simulink model "drivePMSM"  (R2024b)
settings: Solver=VariableStepAuto  StartTime=0.0  StopTime=0.5  MaxStep=1e-3  RelTol=1e-3
undefined symbols (not defined in the file or in its folder): contr_D, contr_Q, contr_Speed, inverter, mot
libraries: simulink x13
settings Model: Creator=giulio  LastModifiedBy=giulio

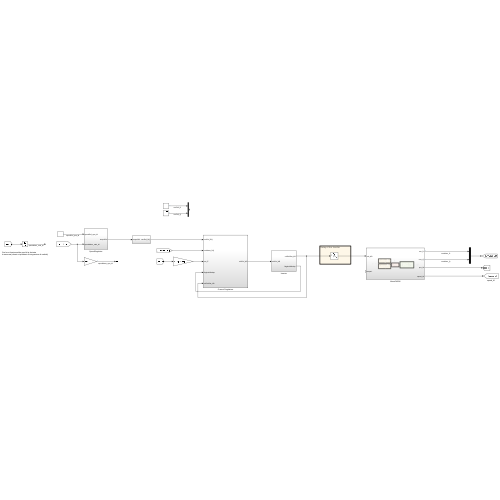
[thumbnail: Simulink's stored preview of the top-level diagram]
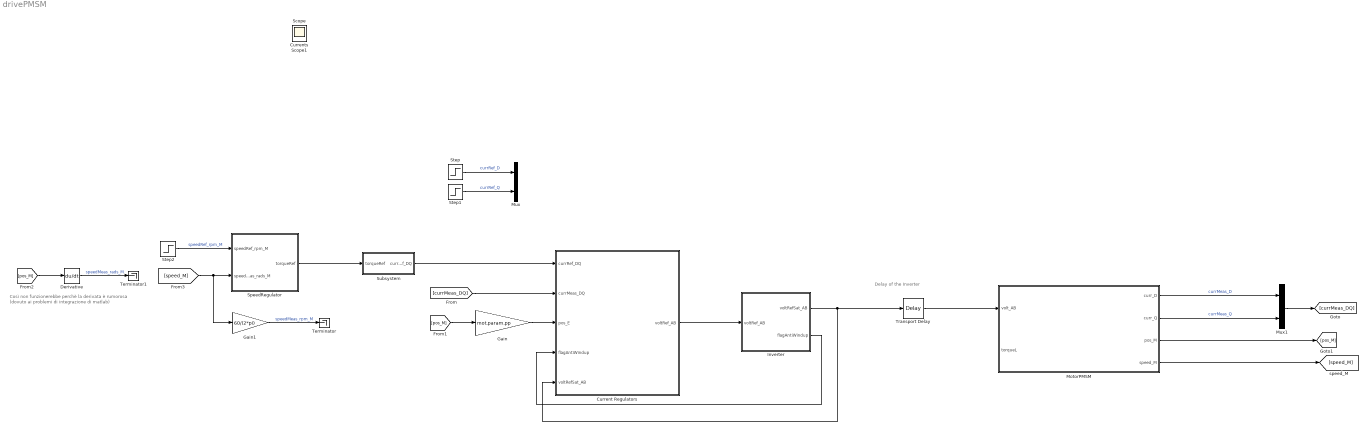
== system drivePMSM ==
  note: Così non funzionerebbe perchè la derivata
      | è rumorosa (dovuto ai problemi di integrazione di matlab)
  note: Delay of the Inverter
  Current Regulators : Subsystem
  Derivative : Derivative
  Gain : Gain  Gain=mot.param.pp
  Gain1 : Gain  Gain=60/(2*pi)
  Inverter : Subsystem
  MotorPMSM : Subsystem
  Mux : Mux  Inputs=2
  Mux1 : Mux  Inputs=2
  SpeedRegulator : Subsystem
  Step : Step  Time=1e-3  SampleTime=0
  Step1 : Step  Time=5e-3  SampleTime=0
  Step2 : Step  Time=0.01  After=0.25*mot.rated.speed_rpm  SampleTime=0
  Subsystem : Subsystem
  Terminator : Terminator
  Terminator1 : Terminator
  Transport Delay : TransportDelay  DelayTime=1.5*inverter.param.timePWM
  Currents : Scope
  Scope : Scope
  Scope1 : Scope
  wires:
  Transport Delay/1 -> MotorPMSM/1(volt_AB)
  Current Regulators/1(voltRef_AB) -> Inverter/1(voltRef_AB)
  Step/1 -> Mux/1  "currRef_D"
  Step1/1 -> Mux/2  "currRef_Q"
  Mux1/1 -> [currMeas_DQ]
  MotorPMSM/1(curr_D) -> Mux1/1  "currMeas_D"
  MotorPMSM/2(curr_Q) -> Mux1/2  "currMeas_Q"
  MotorPMSM/3(pos_M) -> [pos_M]
  [pos_M] -> Gain/1
  Gain/1 -> Current Regulators/3(pos_E)
  Inverter/2(flagAntiWindup) -> Current Regulators/4(flagAntiWindup)
  [currMeas_DQ] -> Current Regulators/2(currMeas_DQ)
  Inverter/1(voltRefSat_AB) -> Current Regulators/5(voltRefSat_AB), Transport Delay/1
  SpeedRegulator/1(torqueRef) -> Subsystem/1(torqueRef)
  Subsystem/1(currRef_DQ) -> Current Regulators/1(currRef_DQ)
  [pos_M] -> Derivative/1
  Step2/1 -> SpeedRegulator/1(speedRef_rpm_M)  "speedRef_rpm_M"
  Gain1/1 -> Terminator/1  "speedMeas_rpm_M"
  MotorPMSM/4(speed_M) -> [speed_M]
  [speed_M] -> Gain1/1, SpeedRegulator/2(speedMeas_rads_M)
  Derivative/1 -> Terminator1/1  "speedMeas_rads_M"

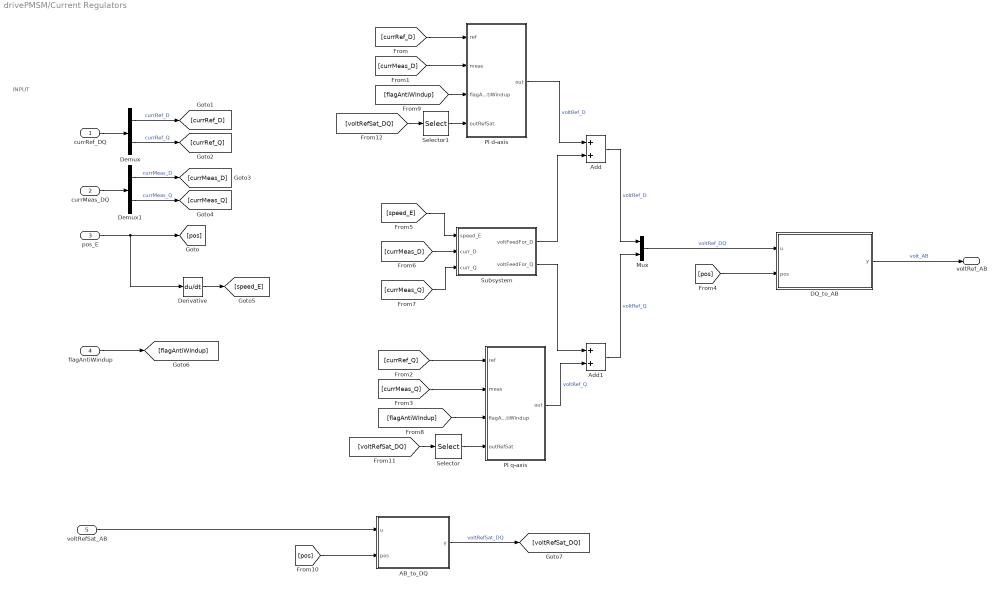
== system drivePMSM/Current Regulators ==
  note: INPUT
  currRef_DQ : Inport
  currMeas_DQ : Inport  Port=2
  pos_E : Inport  Port=3
  flagAntiWindup : Inport  Port=4
  voltRefSat_AB : Inport  Port=5
  AB_to_DQ : MATLAB Function  TreatAsAtomicUnit=on
  Add : Sum
  Add1 : Sum
  DQ_to_AB : MATLAB Function  TreatAsAtomicUnit=on
  Demux : Demux  Outputs=2
  Demux1 : Demux  Outputs=2
  Derivative : Derivative
  Mux : Mux  Inputs=2
  PI d-axis : Subsystem
  PI q-axis : Subsystem
  Selector : Selector  InputPortWidth=2  IndexOptions=Index vector (dialog)  Indices=[2]  OutputSizes=1
  Selector1 : Selector  InputPortWidth=2  IndexOptions=Index vector (dialog)  Indices=[1]  OutputSizes=1
  Subsystem : Subsystem
  voltRef_AB : Outport
  wires:
  Mux/1 -> DQ_to_AB/1(u)  "voltRef_DQ"
  DQ_to_AB/1(y) -> voltRef_AB/1  "volt_AB"
  currRef_DQ/1 -> Demux/1
  Demux/2 -> [currRef_Q]  "currRef_Q"
  currMeas_DQ/1 -> Demux1/1
  Demux1/1 -> [currMeas_D]  "currMeas_D"
  Demux1/2 -> [currMeas_Q]  "currMeas_Q"
  pos_E/1 -> Derivative/1, [pos]
  Demux/1 -> [currRef_D]  "currRef_D"
  [currRef_D] -> PI d-axis/1(ref)
  [currMeas_D] -> PI d-axis/2(meas)
  [currRef_Q] -> PI q-axis/1(ref)
  [currMeas_Q] -> PI q-axis/2(meas)
  [pos] -> DQ_to_AB/2(pos)
  Derivative/1 -> [speed_E]
  [speed_E] -> Subsystem/1(speed_E)
  [currMeas_D] -> Subsystem/2(curr_D)
  [currMeas_Q] -> Subsystem/3(curr_Q)
  PI d-axis/1(out) -> Add/1  "voltRef_D"
  Subsystem/1(voltFeedFor_D) -> Add/2
  PI q-axis/1(out) -> Add1/2  "voltRef_Q"
  Subsystem/2(voltFeedFor_Q) -> Add1/1
  Add1/1 -> Mux/2  "voltRef_Q"
  Add/1 -> Mux/1  "voltRef_D"
  flagAntiWindup/1 -> [flagAntiWIndup]
  [flagAntiWIndup] -> PI q-axis/3(flagAntiWindup)
  [flagAntiWIndup] -> PI d-axis/3(flagAntiWindup)
  voltRefSat_AB/1 -> AB_to_DQ/1(u)
  [pos] -> AB_to_DQ/2(pos)
  AB_to_DQ/1(y) -> [voltRefSat_DQ]  "voltRefSat_DQ"
  [voltRefSat_DQ] -> Selector/1
  Selector/1 -> PI q-axis/4(outRefSat)
  [voltRefSat_DQ] -> Selector1/1
  Selector1/1 -> PI d-axis/4(outRefSat)

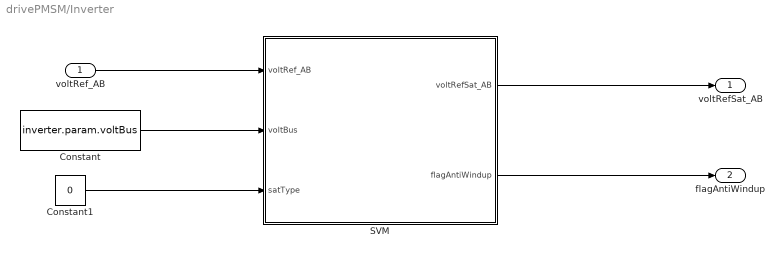
== system drivePMSM/Inverter ==
  voltRef_AB : Inport
  Constant : Constant  Value=inverter.param.voltBus
  Constant1 : Constant  Value=0
  SVM : MATLAB Function  TreatAsAtomicUnit=on
  voltRefSat_AB : Outport
  flagAntiWindup : Outport  Port=2
  wires:
  Constant1/1 -> SVM/3(satType)
  Constant/1 -> SVM/2(voltBus)
  SVM/1(voltRefSat_AB) -> voltRefSat_AB/1
  voltRef_AB/1 -> SVM/1(voltRef_AB)
  SVM/2(flagAntiWindup) -> flagAntiWindup/1

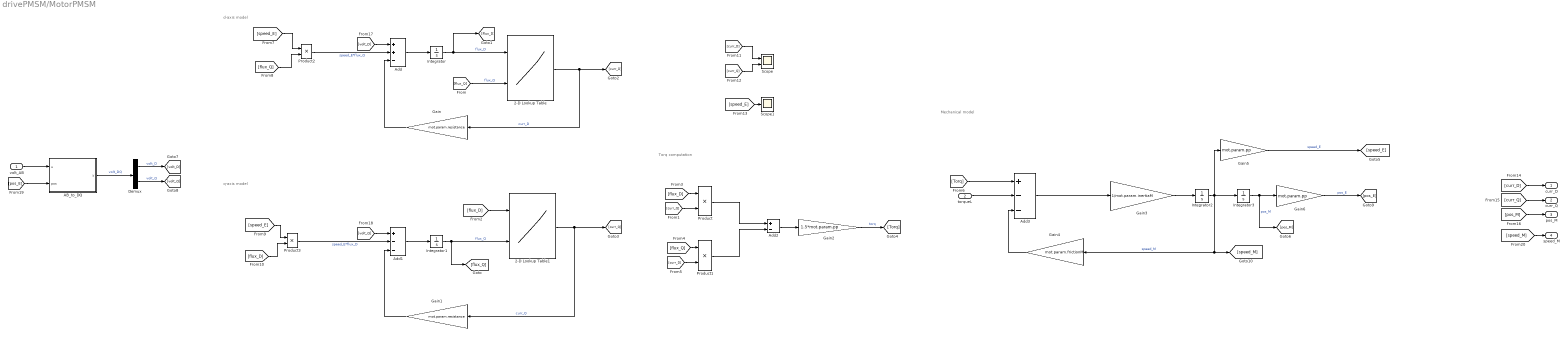
== system drivePMSM/MotorPMSM ==
  note: Mechanical model
  note: Torq computation
  note: d-axis model
  note: q-axis model
  volt_AB : Inport
  torqueL : Inport  Port=2
  2-D Lookup Table : Lookup_n-D  BreakpointsForDimension1=mot.maps.fluxVec_D  BreakpointsForDimension2=mot.maps.fluxVec_Q  Table=mot.maps.currMap_D'  InternalRulePriority=Speed  RndMeth=Simplest
      settings: InputPortMap=u0,u1
  2-D Lookup Table1 : Lookup_n-D  BreakpointsForDimension1=mot.maps.fluxVec_D  BreakpointsForDimension2=mot.maps.fluxVec_Q  Table=mot.maps.currMap_Q'  InternalRulePriority=Speed  RndMeth=Simplest
      settings: InputPortMap=u0,u1
  AB_to_DQ : MATLAB Function  TreatAsAtomicUnit=on
  Add : Sum  Inputs=++-
  Add1 : Sum  Inputs=+--
  Add2 : Sum  Inputs=+-
  Add3 : Sum  Inputs=+--
  Demux : Demux  Outputs=2
  Gain : Gain  Gain=mot.param.resistance
  Gain1 : Gain  Gain=mot.param.resistance
  Gain2 : Gain  Gain=1.5*mot.param.pp
  Gain3 : Gain  Gain=1/mot.param.inertiaM
  Gain4 : Gain  Gain=mot.param.frictionM
  Gain5 : Gain  Gain=mot.param.pp
  Gain6 : Gain  Gain=mot.param.pp
  Integrator : Integrator  InitialCondition=mot.param.fluxPM
  Integrator1 : Integrator
  Integrator2 : Integrator
  Integrator3 : Integrator
  Product{,1..3} (4 alike) : Product
  Scope : Scope  NumInputPorts=2
  Scope1 : Scope
  curr_D : Outport
  curr_Q : Outport  Port=2
  pos_M : Outport  Port=3
  speed_M : Outport  Port=4
  wires:
  [flux_Q] -> Product1/1
  [speed_E] -> Scope1/1
  Integrator3/1 -> [pos_M], Gain6/1  "pos_M"
  Add2/1 -> Gain2/1
  Gain5/1 -> [speed_E]  "speed_E"
  Product/1 -> Add2/1
  Integrator/1 -> [flux_D], 2-D Lookup Table/1  "flux_D"
  Product3/1 -> Add1/2  "speed_E*flux_D"
  Gain4/1 -> Add3/3
  [flux_D] -> Product3/2
  Add/1 -> Integrator/1
  [flux_D] -> 2-D Lookup Table1/1
  Gain/1 -> Add/3
  Integrator2/1 -> Gain5/1, [speed_M], Gain4/1, Integrator3/1  "speed_M"
  Add1/1 -> Integrator1/1
  Gain1/1 -> Add1/3
  [flux_D] -> Product/1
  Add3/1 -> Gain3/1
  [curr_Q] -> Product/2
  Integrator1/1 -> [flux_Q], 2-D Lookup Table1/2  "flux_Q"
  Gain2/1 -> [Torq]  "torq"
  Gain3/1 -> Integrator2/1
  [flux_Q] -> Product2/2
  [curr_D] -> Scope/1
  [curr_Q] -> Scope/2
  torqueL/1 -> Add3/2
  [curr_D] -> Product1/2
  [flux_Q] -> 2-D Lookup Table/2  "flux_Q"
  2-D Lookup Table1/1 -> [curr_Q], Gain1/1  "curr_Q"
  Product2/1 -> Add/2  "speed_E*flux_Q"
  Product1/1 -> Add2/2
  2-D Lookup Table/1 -> [curr_D], Gain/1  "curr_D"
  [Torq] -> Add3/1
  [speed_E] -> Product3/1
  [speed_E] -> Product2/1
  [pos_M] -> pos_M/1
  [curr_Q] -> curr_Q/1
  [curr_D] -> curr_D/1
  AB_to_DQ/1(y) -> Demux/1  "volt_DQ"
  Demux/1 -> [volt_D]  "volt_D"
  Demux/2 -> [volt_Q]  "volt_Q"
  [volt_D] -> Add/1
  [volt_Q] -> Add1/1
  Gain6/1 -> [pos_E]  "pos_E"
  [pos_E] -> AB_to_DQ/2(pos)
  volt_AB/1 -> AB_to_DQ/1(u)
  [speed_M] -> speed_M/1

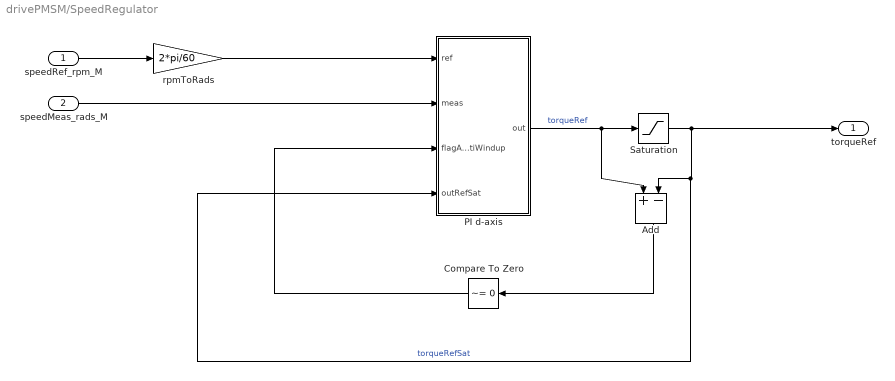
== system drivePMSM/SpeedRegulator ==
  speedRef_rpm_M : Inport
  speedMeas_rads_M : Inport  Port=2
  Add : Sum  Inputs=+-
  Compare To Zero : simulink/Logic and Bit Operations/Compare To Zero  relop=~=  OutDataTypeStr=boolean
  PI d-axis : Subsystem
  Saturation : Saturate  UpperLimit=contr_Speed.param.outMax  LowerLimit=contr_Speed.param.outMin
  rpmToRads : Gain  Gain=2*pi/60
  torqueRef : Outport
  wires:
  rpmToRads/1 -> PI d-axis/1(ref)
  speedRef_rpm_M/1 -> rpmToRads/1
  speedMeas_rads_M/1 -> PI d-axis/2(meas)
  PI d-axis/1(out) -> Add/1, Saturation/1  "torqueRef"
  Saturation/1 -> torqueRef/1, PI d-axis/4(outRefSat), Add/2  "torqueRefSat"
  Add/1 -> Compare To Zero/1
  Compare To Zero/1 -> PI d-axis/3(flagAntiWindup)

== system drivePMSM/Subsystem ==
  torqueRef : Inport
  Constant : Constant  Value=0
  Gain : Gain  Gain=1/(1.5*mot.param.pp*mot.param.fluxPM)
  Mux : Mux  Inputs=2
  currRef_DQ : Outport
  wires:
  torqueRef/1 -> Gain/1
  Constant/1 -> Mux/1
  Gain/1 -> Mux/2
  Mux/1 -> currRef_DQ/1

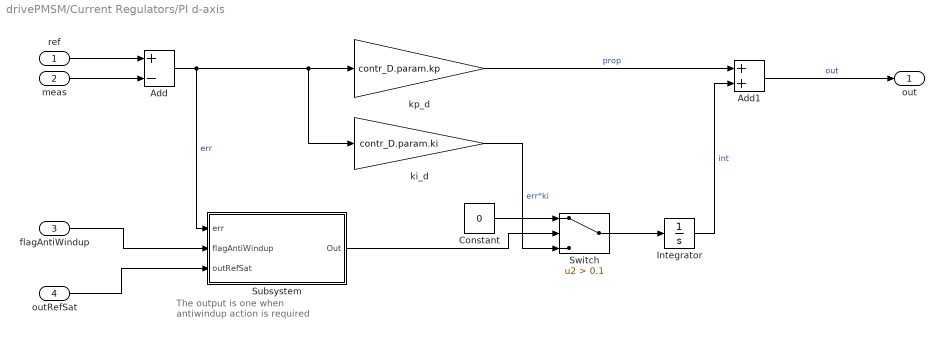
== system drivePMSM/Current Regulators/PI d-axis ==
  note: The output is one when antiwindup action is required
  ref : Inport
  meas : Inport  Port=2
  flagAntiWindup : Inport  Port=3
  outRefSat : Inport  Port=4
  Add : Sum  Inputs=+-
  Add1 : Sum
  Constant : Constant  Value=0
  Integrator : Integrator
  Subsystem : Subsystem
  Switch : Switch  Criteria=u2 > Threshold  Threshold=0.1  SaturateOnIntegerOverflow=off  InputSameDT=off
  ki_d : Gain  Gain=contr_D.param.ki
  kp_d : Gain  Gain=contr_D.param.kp
  out : Outport
  wires:
  Integrator/1 -> Add1/2  "int"
  kp_d/1 -> Add1/1  "prop"
  Add/1 -> Subsystem/1(err), ki_d/1, kp_d/1  "err"
  Add1/1 -> out/1  "out"
  ref/1 -> Add/1
  meas/1 -> Add/2
  flagAntiWindup/1 -> Subsystem/2(flagAntiWindup)
  outRefSat/1 -> Subsystem/3(outRefSat)
  Switch/1 -> Integrator/1
  Constant/1 -> Switch/1
  ki_d/1 -> Switch/3  "err*ki"
  Subsystem/1(Out) -> Switch/2

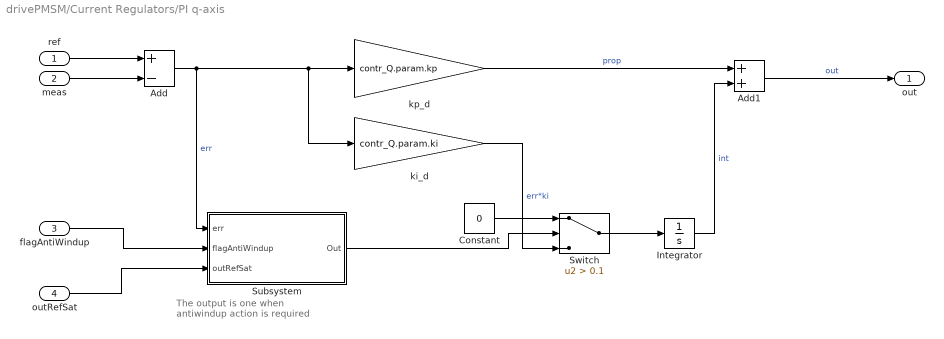
== system drivePMSM/Current Regulators/PI q-axis ==
  note: The output is one when antiwindup action is required
  ref : Inport
  meas : Inport  Port=2
  flagAntiWindup : Inport  Port=3
  outRefSat : Inport  Port=4
  Add : Sum  Inputs=+-
  Add1 : Sum
  Constant : Constant  Value=0
  Integrator : Integrator
  Subsystem : Subsystem
  Switch : Switch  Criteria=u2 > Threshold  Threshold=0.1  SaturateOnIntegerOverflow=off  InputSameDT=off
  ki_d : Gain  Gain=contr_Q.param.ki
  kp_d : Gain  Gain=contr_Q.param.kp
  out : Outport
  wires:
  Integrator/1 -> Add1/2  "int"
  kp_d/1 -> Add1/1  "prop"
  Add/1 -> Subsystem/1(err), ki_d/1, kp_d/1  "err"
  Add1/1 -> out/1  "out"
  ref/1 -> Add/1
  meas/1 -> Add/2
  flagAntiWindup/1 -> Subsystem/2(flagAntiWindup)
  outRefSat/1 -> Subsystem/3(outRefSat)
  Switch/1 -> Integrator/1
  Constant/1 -> Switch/1
  ki_d/1 -> Switch/3  "err*ki"
  Subsystem/1(Out) -> Switch/2

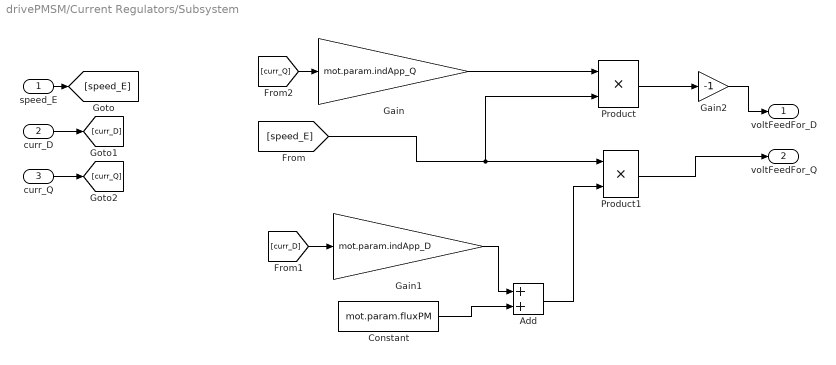
== system drivePMSM/Current Regulators/Subsystem ==
  speed_E : Inport
  curr_D : Inport  Port=2
  curr_Q : Inport  Port=3
  Add : Sum
  Constant : Constant  Value=mot.param.fluxPM
  Gain : Gain  Gain=mot.param.indApp_Q
  Gain1 : Gain  Gain=mot.param.indApp_D
  Gain2 : Gain  Gain=-1
  Product : Product
  Product1 : Product
  voltFeedFor_D : Outport
  voltFeedFor_Q : Outport  Port=2
  wires:
  speed_E/1 -> [speed_E]
  curr_D/1 -> [curr_D]
  curr_Q/1 -> [curr_Q]
  [curr_Q] -> Gain/1
  Gain/1 -> Product/1
  [curr_D] -> Gain1/1
  Constant/1 -> Add/2
  Gain1/1 -> Add/1
  [speed_E] -> Product/2, Product1/1
  Add/1 -> Product1/2
  Product1/1 -> voltFeedFor_Q/1
  Product/1 -> Gain2/1
  Gain2/1 -> voltFeedFor_D/1

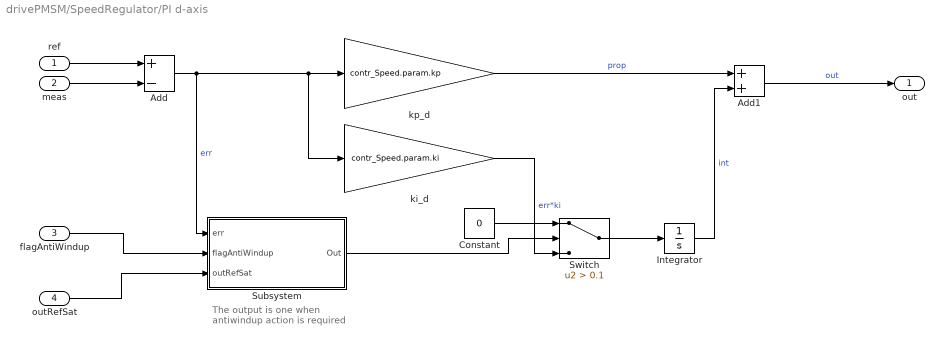
== system drivePMSM/SpeedRegulator/PI d-axis ==
  note: The output is one when antiwindup action is required
  ref : Inport
  meas : Inport  Port=2
  flagAntiWindup : Inport  Port=3
  outRefSat : Inport  Port=4
  Add : Sum  Inputs=+-
  Add1 : Sum
  Constant : Constant  Value=0
  Integrator : Integrator
  Subsystem : Subsystem
  Switch : Switch  Criteria=u2 > Threshold  Threshold=0.1  SaturateOnIntegerOverflow=off  InputSameDT=off
  ki_d : Gain  Gain=contr_Speed.param.ki
  kp_d : Gain  Gain=contr_Speed.param.kp
  out : Outport
  wires:
  Integrator/1 -> Add1/2  "int"
  kp_d/1 -> Add1/1  "prop"
  Add/1 -> Subsystem/1(err), ki_d/1, kp_d/1  "err"
  Add1/1 -> out/1  "out"
  ref/1 -> Add/1
  meas/1 -> Add/2
  flagAntiWindup/1 -> Subsystem/2(flagAntiWindup)
  outRefSat/1 -> Subsystem/3(outRefSat)
  Switch/1 -> Integrator/1
  Constant/1 -> Switch/1
  ki_d/1 -> Switch/3  "err*ki"
  Subsystem/1(Out) -> Switch/2

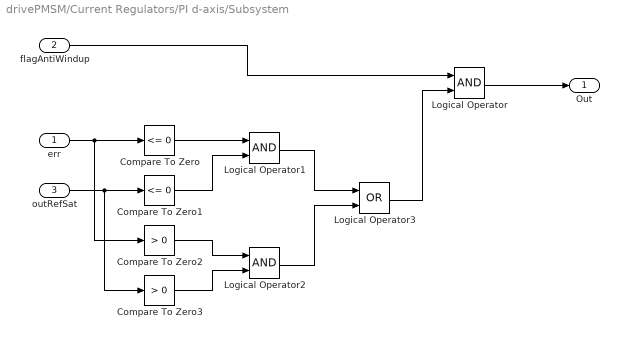
== system drivePMSM/Current Regulators/PI d-axis/Subsystem ==
  err : Inport
  flagAntiWindup : Inport  Port=2
  outRefSat : Inport  Port=3
  Compare To Zero : simulink/Logic and Bit Operations/Compare To Zero  relop=<=  OutDataTypeStr=boolean
  Compare To Zero1 : simulink/Logic and Bit Operations/Compare To Zero  relop=<=  OutDataTypeStr=boolean
  Compare To Zero2 : simulink/Logic and Bit Operations/Compare To Zero  relop=>  OutDataTypeStr=boolean
  Compare To Zero3 : simulink/Logic and Bit Operations/Compare To Zero  relop=>  OutDataTypeStr=boolean
  Logical Operator : Logic  AllPortsSameDT=off  OutDataTypeStr=boolean
  Logical Operator1 : Logic  AllPortsSameDT=off  OutDataTypeStr=boolean
  Logical Operator2 : Logic  AllPortsSameDT=off  OutDataTypeStr=boolean
  Logical Operator3 : Logic  Operator=OR  AllPortsSameDT=off  OutDataTypeStr=boolean
  Out : Outport
  wires:
  Logical Operator/1 -> Out/1
  flagAntiWindup/1 -> Logical Operator/1
  Compare To Zero/1 -> Logical Operator1/1
  Compare To Zero1/1 -> Logical Operator1/2
  outRefSat/1 -> Compare To Zero3/1, Compare To Zero1/1
  err/1 -> Compare To Zero2/1, Compare To Zero/1
  Compare To Zero2/1 -> Logical Operator2/1
  Compare To Zero3/1 -> Logical Operator2/2
  Logical Operator2/1 -> Logical Operator3/2
  Logical Operator1/1 -> Logical Operator3/1
  Logical Operator3/1 -> Logical Operator/2

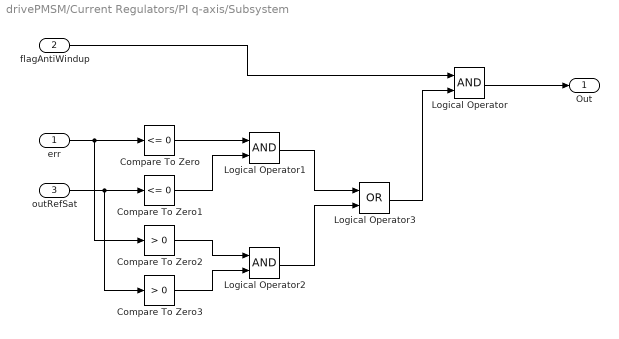
== system drivePMSM/Current Regulators/PI q-axis/Subsystem ==
  err : Inport
  flagAntiWindup : Inport  Port=2
  outRefSat : Inport  Port=3
  Compare To Zero : simulink/Logic and Bit Operations/Compare To Zero  relop=<=  OutDataTypeStr=boolean
  Compare To Zero1 : simulink/Logic and Bit Operations/Compare To Zero  relop=<=  OutDataTypeStr=boolean
  Compare To Zero2 : simulink/Logic and Bit Operations/Compare To Zero  relop=>  OutDataTypeStr=boolean
  Compare To Zero3 : simulink/Logic and Bit Operations/Compare To Zero  relop=>  OutDataTypeStr=boolean
  Logical Operator : Logic  AllPortsSameDT=off  OutDataTypeStr=boolean
  Logical Operator1 : Logic  AllPortsSameDT=off  OutDataTypeStr=boolean
  Logical Operator2 : Logic  AllPortsSameDT=off  OutDataTypeStr=boolean
  Logical Operator3 : Logic  Operator=OR  AllPortsSameDT=off  OutDataTypeStr=boolean
  Out : Outport
  wires:
  Logical Operator/1 -> Out/1
  flagAntiWindup/1 -> Logical Operator/1
  Compare To Zero/1 -> Logical Operator1/1
  Compare To Zero1/1 -> Logical Operator1/2
  outRefSat/1 -> Compare To Zero3/1, Compare To Zero1/1
  err/1 -> Compare To Zero2/1, Compare To Zero/1
  Compare To Zero2/1 -> Logical Operator2/1
  Compare To Zero3/1 -> Logical Operator2/2
  Logical Operator2/1 -> Logical Operator3/2
  Logical Operator1/1 -> Logical Operator3/1
  Logical Operator3/1 -> Logical Operator/2

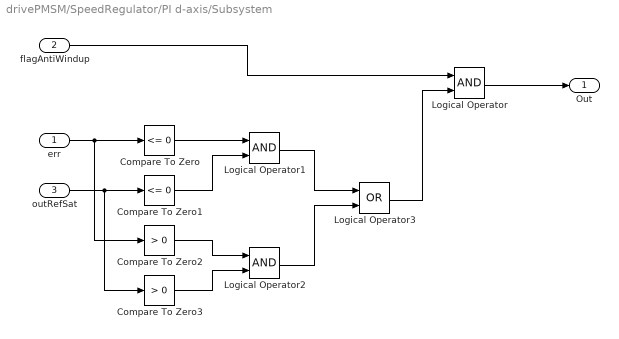
== system drivePMSM/SpeedRegulator/PI d-axis/Subsystem ==
  err : Inport
  flagAntiWindup : Inport  Port=2
  outRefSat : Inport  Port=3
  Compare To Zero : simulink/Logic and Bit Operations/Compare To Zero  relop=<=  OutDataTypeStr=boolean
  Compare To Zero1 : simulink/Logic and Bit Operations/Compare To Zero  relop=<=  OutDataTypeStr=boolean
  Compare To Zero2 : simulink/Logic and Bit Operations/Compare To Zero  relop=>  OutDataTypeStr=boolean
  Compare To Zero3 : simulink/Logic and Bit Operations/Compare To Zero  relop=>  OutDataTypeStr=boolean
  Logical Operator : Logic  AllPortsSameDT=off  OutDataTypeStr=boolean
  Logical Operator1 : Logic  AllPortsSameDT=off  OutDataTypeStr=boolean
  Logical Operator2 : Logic  AllPortsSameDT=off  OutDataTypeStr=boolean
  Logical Operator3 : Logic  Operator=OR  AllPortsSameDT=off  OutDataTypeStr=boolean
  Out : Outport
  wires:
  Logical Operator/1 -> Out/1
  flagAntiWindup/1 -> Logical Operator/1
  Compare To Zero/1 -> Logical Operator1/1
  Compare To Zero1/1 -> Logical Operator1/2
  outRefSat/1 -> Compare To Zero3/1, Compare To Zero1/1
  err/1 -> Compare To Zero2/1, Compare To Zero/1
  Compare To Zero2/1 -> Logical Operator2/1
  Compare To Zero3/1 -> Logical Operator2/2
  Logical Operator2/1 -> Logical Operator3/2
  Logical Operator1/1 -> Logical Operator3/1
  Logical Operator3/1 -> Logical Operator/2

== matlab function drivePMSM/MotorPMSM/AB_to_DQ ==
  data: u input; y output; pos input
function y = AB2DQ(u, pos)
% u = 2x1 vector
% y = 2x1 vector 
% pos = position in rad 

% Transformation matrix 
T_AB2DQ = [cos(pos) sin(pos);...
           -sin(pos) cos(pos)];

% Get output
y = T_AB2DQ * u ;

== matlab function drivePMSM/Inverter/SVM ==
  data: voltRef_AB input; voltRefSat_AB output; voltBus input; satType input; inverter parameter; flagAntiWindup output
function [voltRefSat_AB, flagAntiWindup] = fcn(voltRef_AB,voltBus,satType,inverter)
%satType = 0 -> circular saturation 
%satType = 1 -> hexagonal saturation 

Tpwm = inverter.param.timePWM;
%%%
%Reset flag antiwindup
flagAntiWindup = 0;
%% Circular saturation 
voltRefMag_AB = sqrt(voltRef_AB(1)^2+voltRef_AB(2)^2);
voltBus_sqrt3 = voltBus / sqrt(3);

if ((satType == 0) && (voltRefMag_AB > voltBus_sqrt3))
    %Circular saturation 
    k_sat = voltBus_sqrt3 / voltRefMag_AB;
    voltRefSat_AB = voltRef_AB * k_sat;
    %rise up antiwindup flag
    flagAntiWindup = 1;
else
    voltRefSat_AB = voltRef_AB;
end

%% Sector identification
if (voltRefSat_AB(2) >= 0) %1,2 o 3 sector
    if(voltRefSat_AB(1) >= 0) %1 o 2 sector
        if(voltRefSat_AB(1)*sqrt(3) > voltRefSat_AB(2)) % 1 sector
            m = 1;
        else 
            m = 2;
        end
    else 
        if(voltRefSat_AB(1)*(-sqrt(3)) <= voltRefSat_AB(2))
            m = 2;
        else 
            m = 3;
        end

    end
else % 4,5,6 sector 
    if(voltRefSat_AB(1) < 0) %4 o 5 sector
        if(voltRefSat_AB(1)*-sqrt(3) > -voltRefSat_AB(2))
            m = 4;
        else 
            m = 5;
        end
    else 
        if(voltRefSat_AB(1)*(sqrt(3)) <= -voltRefSat_AB(2))
            m = 5;
        else 
            m = 6;
        end

    end

end

%% Time vector application

k_T = sqrt(3) * Tpwm/voltBus;


T1 =  k_T * (voltRefSat_AB(1) * sin(m*pi/3) - voltRefSat_AB(2) * cos(m * pi/3));
T2 =  k_T * (-voltRefSat_AB(1) * sin((m-1)*pi/3) + voltRefSat_AB(2) * cos((m-1) * pi/3));

% get null vector time 
T0 = Tpwm - T1 - T2;


%% Check hexagonal saturation

if(T0 < 0)
    % hexagonal saturation 
    k_sat = Tpwm/(T1+T2);
    T1 = T1 * k_sat;
    T2 = T2 * k_sat;
    %saturate voltages 
    voltRefSat_AB = voltRefSat_AB*k_sat;
    %rise up antiwindup flag
    flagAntiWindup = 1;
end

== matlab function drivePMSM/Current Regulators/DQ_to_AB ==
  data: u input; y output; pos input
function y = DQ2AB(u, pos)
% u = 2x1 vector
% y = 2x1 vector 
% pos = position in rad 

% Transformation matrix 
T_DQ2AB = [cos(pos) -sin(pos);...
           sin(pos) cos(pos)];

% Get output
y = T_DQ2AB * u ;

== matlab function drivePMSM/Current Regulators/AB_to_DQ ==
  data: u input; y output; pos input
function y = AB2DQ(u, pos)
% u = 2x1 vector
% y = 2x1 vector 
% pos = position in rad 

% Transformation matrix 
T_AB2DQ = [cos(pos) sin(pos);...
           -sin(pos) cos(pos)];

% Get output
y = T_AB2DQ * u ;
